simulink model "truckt_ROS_mpc_8dof_2020a"  (R2020a)
settings: Solver=FixedStepAuto  StartTime=0.0  StopTime=40  FixedStep=0.001  RelTol=1e-3
model workspace (MAT data in the model file):
  Logfile_Data_Object : robotics.ros.BagSelection (value not decoded)
  Logfile_Path = 'D:\robotruck_school\robotruck_school\ws\2025-05-22-09-01-20-filter.bag'
  Logfile_Playback_Duration = nan
  Logfile_Playback_Offset = nan
undefined symbols (not defined in the file): Ax, Ay, Header, SteeringAngle, Vx, Vy, WheelSpeedFl, WheelSpeedFr, X, Y, Yaw
libraries: neural x31, robotlib x5, simulink x2, Solver_SF x1
(part 2 of 2)

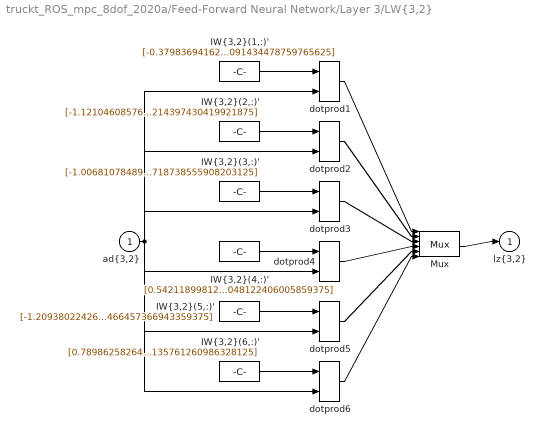
== system truckt_ROS_mpc_8dof_2020a/Feed-Forward Neural Network/Layer 3/LW{3,2} ==
  "ad{3,2}" : Inport  PortDimensions=12  SampleTime=0.0005
      mask Display: e = 0.06;c1 = [120 230 180]/255;c2 = ([120 230 180]+0)/(256+128);c3 = ([120 230 180]+128)/(256+128);patch([0 1 1 0],[0 0 1 1],c1);patch([0 1 1 1-e 1-e 0+e],[0 0 1 1-e 0+e 0+e],c2);patch([0 0 1 1-e 0+e 0+e],[0 1 1 1-e 1-e 0+e],c3);plot([0 1 1 0 0],[0 0 1 1 0]);
  "IW{3,2}(1,:)'" : Constant  Value=[-0.379836941626675306249438790473504923284053802490234375;-0.98830696768600823087780327114160172641277313232421875;-1.5284090636957869957512912151287309825420379638671875;1.9919333469003437375732801228878088295459747314453125;0.11440319696900287660401573930357699282467365264892578125;0.97683677390134493467854781556525267660617828369140625;-0.53691041996622679288719837131793610751628875732421875;0.7817290187824041947095565774361602962017059326171875;1.1256138255462462272049606326618231832981109619140625;-0.1647439148723537638563385598899913020431995391845703125;-0.378423515686045153216809922014363110065460205078125;0.7466735721545367798768211287097074091434478759765625]
      mask Display: e = 0.06;c1 = [120 150 230]/255;c2 = ([120 150 230]+0)/383;c3 = ([120 150 230]+128)/383;patch([0 1 1 0],[0 0 1 1],c1);patch([0 1 1 1-e 1-e 0+e],[0 0 1 1-e 0+e 0+e],c2);patch([0 0 1 1-e 0+e 0+e],[0 1 1 1-e 1-e 0+e],c3);plot([0 1 1 0 0],[0 0 1 1 0]);disp('weights');
  "IW{3,2}(2,:)'" : Constant  Value=[-1.1210460857616471042064176799613051116466522216796875;-0.7419552767831680828436446972773410379886627197265625;0.53241483779089959771368967267335392534732818603515625;-1.1766399501868891608324929620721377432346343994140625;-0.09463379116641357224892772137536667287349700927734375;-1.0754088453349235354750135229551233351230621337890625;2.058569179005649285585377583629451692104339599609375;0.1845364435258407820317216874173027463257312774658203125;-0.14125166896967578100685614117537625133991241455078125;0.366140353791848782716300547690480016171932220458984375;0.84467990539439685715450423231231980025768280029296875;-0.82157153453835440881647400601650588214397430419921875]
      mask Display: e = 0.06;c1 = [120 150 230]/255;c2 = ([120 150 230]+0)/383;c3 = ([120 150 230]+128)/383;patch([0 1 1 0],[0 0 1 1],c1);patch([0 1 1 1-e 1-e 0+e],[0 0 1 1-e 0+e 0+e],c2);patch([0 0 1 1-e 0+e 0+e],[0 1 1 1-e 1-e 0+e],c3);plot([0 1 1 0 0],[0 0 1 1 0]);disp('weights');
  "IW{3,2}(3,:)'" : Constant  Value=[-1.006810784893824806118800552212633192539215087890625;0.95192185992205147204714421604876406490802764892578125;0.9298205533296572955492820256040431559085845947265625;1.0149920449997242855033618980087339878082275390625;1.066763892614790876223196391947567462921142578125;-1.5026328411580152089044304375420324504375457763671875;-0.2887488368487722834032638274948112666606903076171875;-0.274322719613227683499445674897287972271442413330078125;-1.1607228091908494693740294678718782961368560791015625;-1.164336171214203741186565821408294141292572021484375;-1.2075793320365004746008708025328814983367919921875;0.2939677320845259789194869881612248718738555908203125]
      mask Display: e = 0.06;c1 = [120 150 230]/255;c2 = ([120 150 230]+0)/383;c3 = ([120 150 230]+128)/383;patch([0 1 1 0],[0 0 1 1],c1);patch([0 1 1 1-e 1-e 0+e],[0 0 1 1-e 0+e 0+e],c2);patch([0 0 1 1-e 0+e 0+e],[0 1 1 1-e 1-e 0+e],c3);plot([0 1 1 0 0],[0 0 1 1 0]);disp('weights');
  "IW{3,2}(4,:)'" : Constant  Value=[0.5421189981226792742319275930640287697315216064453125;0.83648451003989998664422955698682926595211029052734375;0.034333862316999884389812081053605652414262294769287109375;-0.9791461692120773108172215870581567287445068359375;-1.4778178014431155862240530041162855923175811767578125;-1.259084079819064783123394590802490711212158203125;-1.2322649693903908740821862011216580867767333984375;-1.1568566233331540882289800720172934234142303466796875;0.675147602978973804255247159744612872600555419921875;0.943289992486696871054618895868770778179168701171875;0.302252716047769764973196515711606480181217193603515625;-0.75126287076459374869585872147581540048122406005859375]
      mask Display: e = 0.06;c1 = [120 150 230]/255;c2 = ([120 150 230]+0)/383;c3 = ([120 150 230]+128)/383;patch([0 1 1 0],[0 0 1 1],c1);patch([0 1 1 1-e 1-e 0+e],[0 0 1 1-e 0+e 0+e],c2);patch([0 0 1 1-e 0+e 0+e],[0 1 1 1-e 1-e 0+e],c3);plot([0 1 1 0 0],[0 0 1 1 0]);disp('weights');
  "IW{3,2}(5,:)'" : Constant  Value=[-1.209380224263462810796454505180008709430694580078125;-1.2418346512138871418073904351331293582916259765625;-1.093742864610391052337945438921451568603515625;1.106517387891877479688673702185042202472686767578125;0.0310794670219283648837649280949335661716759204864501953125;0.66536658754302890894649635811219923198223114013671875;-0.442636928145275387880275275165331549942493438720703125;-0.98844127648950197428945330102578736841678619384765625;-1.08142840752187918695881307939998805522918701171875;-0.0222259212521214687130477472010170458815991878509521484375;1.0011391938590052941293606636463664472103118896484375;0.9845721918984080556214166790596209466457366943359375]
      mask Display: e = 0.06;c1 = [120 150 230]/255;c2 = ([120 150 230]+0)/383;c3 = ([120 150 230]+128)/383;patch([0 1 1 0],[0 0 1 1],c1);patch([0 1 1 1-e 1-e 0+e],[0 0 1 1-e 0+e 0+e],c2);patch([0 0 1 1-e 0+e 0+e],[0 1 1 1-e 1-e 0+e],c3);plot([0 1 1 0 0],[0 0 1 1 0]);disp('weights');
  "IW{3,2}(6,:)'" : Constant  Value=[0.7898625826477292388716477944399230182170867919921875;-1.11184879157876803645876861992292106151580810546875;0.64732700347357685632943002929096110165119171142578125;1.185066102343848459810260465019382536411285400390625;0.3984215957234378269191665822290815412998199462890625;1.4082692791027484613408660152344964444637298583984375;0.43243315306744900539115405990742146968841552734375;-0.9736958147140117869611231071758083999156951904296875;0.8420544715029658622285069213830865919589996337890625;0.391210183683046330838095627768780104815959930419921875;-0.1416235594917918394486378019792027771472930908203125;0.97683922117288546349556099812616594135761260986328125]
      mask Display: e = 0.06;c1 = [120 150 230]/255;c2 = ([120 150 230]+0)/383;c3 = ([120 150 230]+128)/383;patch([0 1 1 0],[0 0 1 1],c1);patch([0 1 1 1-e 1-e 0+e],[0 0 1 1-e 0+e 0+e],c2);patch([0 0 1 1-e 0+e 0+e],[0 1 1 1-e 1-e 0+e],c3);plot([0 1 1 0 0],[0 0 1 1 0]);disp('weights');
  Mux : Mux  Inputs=6
      mask Display: e = 0.06;c1 = [120 150 230]/255;c2 = ([120 150 230]+0)/383;c3 = ([120 150 230]+128)/383;patch([0 1 1 0],[0 0 1 1],c1);patch([0 1 1 1-e 1-e 0+e],[0 0 1 1-e 0+e 0+e],c2);patch([0 0 1 1-e 0+e 0+e],[0 1 1 1-e 1-e 0+e],c3);plot([0 1 1 0 0],[0 0 1 1 0]);disp('Mux');
  dotprod{1..6} (6 alike) : neural/Weight Functions/dotprod
  "lz{3,2}" : Outport
      mask Display: e = 0.06;c1 = [120 230 180]/255;c2 = ([120 230 180]+0)/(256+128);c3 = ([120 230 180]+128)/(256+128);patch([0 1 1 0],[0 0 1 1],c1);patch([0 1 1 1-e 1-e 0+e],[0 0 1 1-e 0+e 0+e],c2);patch([0 0 1 1-e 0+e 0+e],[0 1 1 1-e 1-e 0+e],c3);plot([0 1 1 0 0],[0 0 1 1 0]);
  wires:
  "IW{3,2}(1,:)'"/1 -> dotprod1/1
  "ad{3,2}"/1 -> dotprod1/2, dotprod2/2, dotprod3/2, dotprod4/2, dotprod5/2, dotprod6/2
  dotprod1/1 -> Mux/1
  "IW{3,2}(2,:)'"/1 -> dotprod2/1
  dotprod2/1 -> Mux/2
  "IW{3,2}(3,:)'"/1 -> dotprod3/1
  dotprod3/1 -> Mux/3
  "IW{3,2}(4,:)'"/1 -> dotprod4/1
  dotprod4/1 -> Mux/4
  "IW{3,2}(5,:)'"/1 -> dotprod5/1
  dotprod5/1 -> Mux/5
  "IW{3,2}(6,:)'"/1 -> dotprod6/1
  dotprod6/1 -> Mux/6
  Mux/1 -> "lz{3,2}"/1

== system truckt_ROS_mpc_8dof_2020a/Feed-Forward Neural Network/Layer 4/Delays 1 ==
  "p{4}" : Inport  PortDimensions=6  SampleTime=0.0005
      mask Display: e = 0.06;c1 = [120 230 180]/255;c2 = ([120 230 180]+0)/(256+128);c3 = ([120 230 180]+128)/(256+128);patch([0 1 1 0],[0 0 1 1],c1);patch([0 1 1 1-e 1-e 0+e],[0 0 1 1-e 0+e 0+e],c2);patch([0 0 1 1-e 0+e 0+e],[0 1 1 1-e 1-e 0+e],c3);plot([0 1 1 0 0],[0 0 1 1 0]);
  mux : Mux  Inputs=1
      mask Display: e = 0.06;c1 = [120 150 230]/255;c2 = ([120 150 230]+0)/383;c3 = ([120 150 230]+128)/383;patch([0 1 1 0],[0 0 1 1],c1);patch([0 1 1 1-e 1-e 0+e],[0 0 1 1-e 0+e 0+e],c2);patch([0 0 1 1-e 0+e 0+e],[0 1 1 1-e 1-e 0+e],c3);plot([0 1 1 0 0],[0 0 1 1 0]);disp('Mux')
  "pd{4,3}" : Outport
      mask Display: e = 0.06;c1 = [120 230 180]/255;c2 = ([120 230 180]+0)/(256+128);c3 = ([120 230 180]+128)/(256+128);patch([0 1 1 0],[0 0 1 1],c1);patch([0 1 1 1-e 1-e 0+e],[0 0 1 1-e 0+e 0+e],c2);patch([0 0 1 1-e 0+e 0+e],[0 1 1 1-e 1-e 0+e],c3);plot([0 1 1 0 0],[0 0 1 1 0]);
  wires:
  "p{4}"/1 -> mux/1
  mux/1 -> "pd{4,3}"/1

== system truckt_ROS_mpc_8dof_2020a/Feed-Forward Neural Network/Layer 4/LW{4,3} ==
  "ad{4,3}" : Inport  PortDimensions=6  SampleTime=0.0005
      mask Display: e = 0.06;c1 = [120 230 180]/255;c2 = ([120 230 180]+0)/(256+128);c3 = ([120 230 180]+128)/(256+128);patch([0 1 1 0],[0 0 1 1],c1);patch([0 1 1 1-e 1-e 0+e],[0 0 1 1-e 0+e 0+e],c2);patch([0 0 1 1-e 0+e 0+e],[0 1 1 1-e 1-e 0+e],c3);plot([0 1 1 0 0],[0 0 1 1 0]);
  "IW{4,3}(1,:)'" : Constant  Value=[1.0365086789271795719713509242865256965160369873046875;-0.07770699028544313102795371150932624004781246185302734375;-0.9449999401189803638345665603992529213428497314453125;0.1511782678576858440777641590102575719356536865234375;0.25449790728671828343721017517964355647563934326171875;-1.6818672952565700828841954717063345015048980712890625]
      mask Display: e = 0.06;c1 = [120 150 230]/255;c2 = ([120 150 230]+0)/383;c3 = ([120 150 230]+128)/383;patch([0 1 1 0],[0 0 1 1],c1);patch([0 1 1 1-e 1-e 0+e],[0 0 1 1-e 0+e 0+e],c2);patch([0 0 1 1-e 0+e 0+e],[0 1 1 1-e 1-e 0+e],c3);plot([0 1 1 0 0],[0 0 1 1 0]);disp('weights');
  Mux : Mux  Inputs=1
      mask Display: e = 0.06;c1 = [120 150 230]/255;c2 = ([120 150 230]+0)/383;c3 = ([120 150 230]+128)/383;patch([0 1 1 0],[0 0 1 1],c1);patch([0 1 1 1-e 1-e 0+e],[0 0 1 1-e 0+e 0+e],c2);patch([0 0 1 1-e 0+e 0+e],[0 1 1 1-e 1-e 0+e],c3);plot([0 1 1 0 0],[0 0 1 1 0]);disp('Mux');
  dotprod1 : neural/Weight Functions/dotprod
  "lz{4,3}" : Outport
      mask Display: e = 0.06;c1 = [120 230 180]/255;c2 = ([120 230 180]+0)/(256+128);c3 = ([120 230 180]+128)/(256+128);patch([0 1 1 0],[0 0 1 1],c1);patch([0 1 1 1-e 1-e 0+e],[0 0 1 1-e 0+e 0+e],c2);patch([0 0 1 1-e 0+e 0+e],[0 1 1 1-e 1-e 0+e],c3);plot([0 1 1 0 0],[0 0 1 1 0]);
  wires:
  "IW{4,3}(1,:)'"/1 -> dotprod1/1
  "ad{4,3}"/1 -> dotprod1/2
  dotprod1/1 -> Mux/1
  Mux/1 -> "lz{4,3}"/1

== matlab function truckt_ROS_mpc_8dof_2020a/Speed PID controller/MATLAB Function1 ==
  data: u input; th output; b output
function [th, b]= fcn(u)

if u >= 0
    th=u;
    b=0;
elseif u<0
    th=0;
    b=u;
else
    th = 0;
    b = 0;
end

== matlab function truckt_ROS_mpc_8dof_2020a/MPC Controller/MPC controller ==
  data: Xo input; steer output; Yo input; Yaw input; Yr input; V input; Vy input; Yaw_rate input; Yawr input
function steer = fcn(Xo, Yo, Yaw, Yr, V, Vy, Yaw_rate, Yawr)
x_k = [Yo-Yr;
       Yaw - Yawr;
       0;
       0]; %后两维可以编写一个误差获取的模块加在前面
N = 100;
%定义系统矩阵
q=[10,10,1,1];
Q = diag(q);
R = 1;
T = 0.001;

kf=140000;
km=120000;
kr=120000;
m=61000;
Iz=23665;
a=2.2;
b=2;
c=3.9;

if V <= 0.5
    V = 0.5;
end

tildeA = [1 V*T           T                              0                           ;
          0 1             0                              T                           ;
          0 0             1-T*(kf+km+kr)/(m*V)           -T*(a*kf-b*km-c*kr)/(m*V)-V*T    ;
          0 0             -T*(a*kf-b*km-c*kr)/(Iz*V)      1-T*(a*a*kf+b*b*km+c*c*kr)/(Iz*V)];

tildeB = [0;
          0;
          T*kf/m;
          T*a*kf/Iz];


n = size(tildeA,1);
p = size(tildeB,2);

Psi = zeros(N*n, n);
Theta = zeros(N*n,N*p);
tmp=eye(n);


for i = 1:N
    rows = (i-1)*n+(1:n);
    if i == 1
        Theta(rows, 1:p) = tmp*tildeB;
    else
        Theta(rows, :) = [tmp*tildeB, Theta(rows-n, 1:end-p)];
    end
    tmp = tildeA*tmp;
    Psi(rows,:) = tmp;
end

Q_bar = kron(eye(N),Q);
R_bar = kron(eye(N),R);

E = Theta'*Q_bar*Psi;
H = Theta'*Q_bar*Theta + R_bar;
error = Psi*x_k;
% print(size(error))
U_k = zeros(N*p, 1);
U_k = -H^-1*E*x_k;

steer = U_k(1:p,1);%1:p



% function steer = fcn(Xo, Yo ,Yaw, Yr, V, deltar)
% x_k = [Yo-Yr;
%         Yaw;
%         0];
% N = 100;
% %定义系统矩阵
% Q = [30 0 0;
%      0 20 0;
%      0 0 1];
% R = 0.5;
% T = 0.001;
% l=6.2;
% tildeA = [1 T*V*cos(deltar) 0;
%           0     1 T*V/(l*cos(deltar)^2);
%           0     0       -(1/0.2) + 1];
% 
% tildeB = [0;
%           0;
%           0.0005/0.2];
% 
% n = size(tildeA,1);
% p = size(tildeB,2);
% 
% Psi = zeros(N*n, n);
% Theta = zeros(N*n,N*p);
% tmp=eye(n);
% 
% 
% for i = 1:N
%     rows = (i-1)*n+(1:n);
%     if i == 1
%         Theta(rows, 1:p) = tmp*tildeB;
%     else
%         Theta(rows, :) = [tmp*tildeB, Theta(rows-n, 1:end-p)];
%     end
%     tmp = tildeA*tmp;
%     Psi(rows,:) = tmp;
% end
% 
% Q_bar = kron(eye(N),Q);
% R_bar = kron(eye(N),R);
% 
% E = Theta'*Q_bar*Psi;
% H = Theta'*Q_bar*Theta + R_bar;
% 
% U_k = zeros(N*p, 1);
% U_k = -H^-1*E*x_k;
% 
% steer = U_k(1,1);%1:p

== matlab function truckt_ROS_mpc_8dof_2020a/Noise Generator ==
  data: steer input; esteer_sin_noise output; yaw input; speed input
function esteer_sin_noise = fcn(steer,yaw,speed)

esteer_sin_noise = 5*sin(0.11*steer)*sin(0.05*(yaw-51)) ...
*sin(1.18*speed)+0.15*sin(3.11*steer)*sin(1.05*(yaw-51));

== matlab function truckt_ROS_mpc_8dof_2020a/MPC Controller/MATLAB Function1 ==
  data: x input; y output
function y = fcn(x)
r1=0.096*(x-60)-1.2;
r2=0.096*(x-120)-1.2;
dm1=25;
dm2=25;
dn1=3.6;
dn2=3.6;
y = dn1/2*(1+tanh(r1))-dn2/2*(1+tanh(r2));

== matlab function truckt_ROS_mpc_8dof_2020a/MPC Controller/MATLAB Function2 ==
  data: x input; yaw output
function yaw = fcn(x)
r1=0.096*(x-60)-1.2;
r2=0.096*(x-120)-1.2;
dm1=25;
dm2=25;
dn1=3.6;
dn2=3.6;
yaw = atan(dn1*(1/cosh(r1))^2*(1.2/dm1)-dn2*(1/cosh(r2))^2*(1.2/dm2));

== matlab function truckt_ROS_mpc_8dof_2020a/MPC Controller/MATLAB Function ==
  data: t input; u input; y output
function y = fcn(t, u)
if t <= 0.1
    u=0.000001;
end

if u >= 40
    u=40;
end

if u <= -40
    u=-40;
end

y = u;

== matlab function truckt_ROS_mpc_8dof_2020a/数学模型 ==
  data: x input; u input; dotx output; V input
function dotx = fcn(x,u,V)

kf=140000;
km=120000;
kr=120000;
m=61000;
Iz=650000;
a=2.2;
b=2;
c=3.9;

if V <= 0.5
    V = 0.5;
end

A = [0 V           1                              0                           ;
     0 0           0                              1                           ;
     0 0           -(kf+km+kr)/(m*V)               -(a*kf-b*km-c*kr)/(m*V)-V    ;
     0 0           -(a*kf-b*km-c*kr)/(Iz*V)        -(a*a*kf+b*b*km+c*c*kr)/(Iz*V)];

B = [0;
     0;
     kf/m;
     a*kf/Iz];

dotx = A*x+B*u;

== matlab function truckt_ROS_mpc_8dof_2020a/数学模型1 ==
  data: x input; u input; xdot output; V input
function xdot = fcn(x,u,V)
l=6.2;

xdot = [sin(x(2))*V;
        (tan(u)/l)*V];

== matlab function truckt_ROS_mpc_8dof_2020a/MATLAB Function ==
  data: vx input; yaw input; vy input; y output
function y = fcn(vx, yaw, vy)
R = [cos(yaw), -sin(yaw);
     sin(yaw),  cos(yaw)];

% 转换到全局坐标系
v_global = R * [vx; vy];
y = v_global;

== matlab function truckt_ROS_mpc_8dof_2020a/MATLAB Function1 ==
  data: ax input; yaw input; ay input; y output
function y = fcn(ax, yaw, ay)
R = [cos(yaw), -sin(yaw);
     sin(yaw),  cos(yaw)];

% 转换到全局坐标系
a_global = R * [ax; ay];
y = a_global;
